simulink model "accelerationTestUnit"  (R2015b)
settings: Solver=FixedStepAuto  StartTime=0.0  StopTime=inf  RelTol=1e-3
undefined symbols (not defined in the file): DiscIntNeverNeededParam
libraries: frdmtfcshieldlib x2, freescalecupcompanionlib x1, simulink_extras x1
settings Model: SimulationMode=external  ExtModeTrigDuration=125  ExtModeArchiveMode=auto  ExtModeArchiveFileName=data-measures  ExtModeArchiveDirName=C:\Users\ap6515\Desktop\Group Project  ExtModeAddSuffixToVar=on  ExtModeWriteAllDataToWs=on  Creator=DM1515  LastModifiedBy=ap6515
settings OptimizationCC: OptimizeModelRefInitCode=on  LifeSpan=1  MaxStackSize=64
settings HardwareCC: ProdBitPerPointer=32  ProdLargestAtomicInteger=Long  ProdLargestAtomicFloat=Double  ProdWordSize=32  ProdHWDeviceType=ARM Compatible->ARM Cortex
settings RTWCC: SystemTargetFile=ert.tlc  TemplateMakefile=ert_default_tmf  Description=Embedded Coder  Toolchain=GNU Tools for ARM Embedded Processors
settings CodeAppCC: IgnoreCustomStorageClasses=off

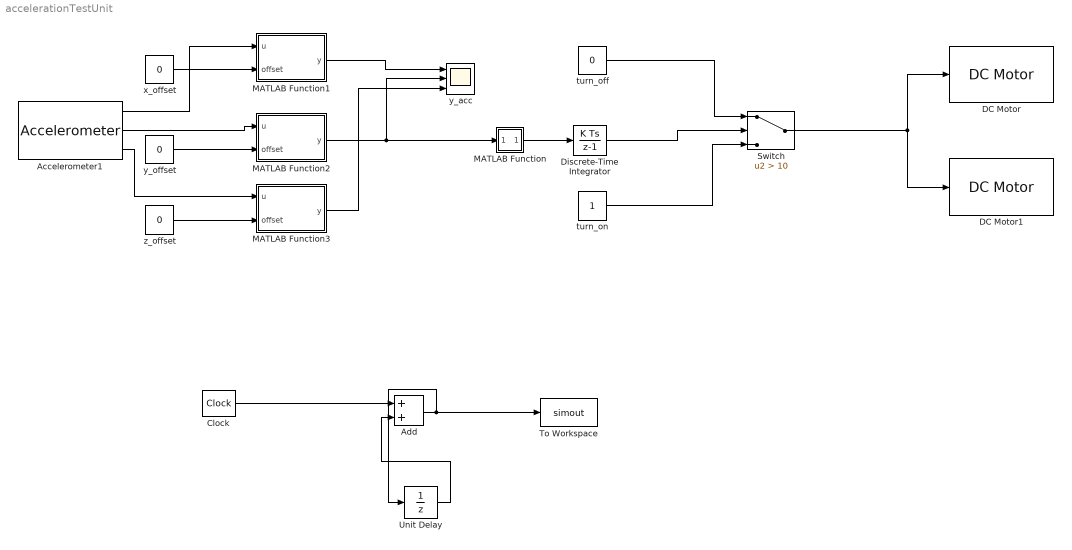
== system accelerationTestUnit ==
  Accelerometer1 : freescalecupcompanionlib/Accelerometer  SampleTime=-1
  Add : Sum
  Clock : simulink_extras/Flip Flops/Clock  period=2
  DC Motor : frdmtfcshieldlib/DC Motor  WhichMotor=A
  DC Motor1 : frdmtfcshieldlib/DC Motor  WhichMotor=B
  Discrete-Time Integrator : DiscreteIntegrator  InitialConditionSetting=State (most efficient)  SampleTime=-1  ICPrevOutput=DiscIntNeverNeededParam  ICPrevScaledInput=DiscIntNeverNeededParam
  MATLAB Function : MATLAB Function  TreatAsAtomicUnit=on
  MATLAB Function1 : MATLAB Function  TreatAsAtomicUnit=on
  MATLAB Function2 : MATLAB Function  TreatAsAtomicUnit=on
  MATLAB Function3 : MATLAB Function  TreatAsAtomicUnit=on
  Switch : Switch  Criteria=u2 > Threshold  Threshold=10
  To Workspace : ToWorkspace  VariableName=simout  SaveFormat=Structure With Time  SampleTime=-1
  Unit Delay : UnitDelay  SampleTime=-1
  turn_off : Constant  Value=0  SampleTime=-1
  turn_on : Constant  SampleTime=-1
  x_offset : Constant  Value=0  SampleTime=-1
  y_acc : Scope  NumInputPorts=3
  y_offset : Constant  Value=0  SampleTime=-1
  z_offset : Constant  Value=0  SampleTime=-1
  wires:
  Switch/1 -> DC Motor/1, DC Motor1/1
  turn_off/1 -> Switch/1
  turn_on/1 -> Switch/3
  Discrete-Time Integrator/1 -> Switch/2
  MATLAB Function/1(y) -> Discrete-Time Integrator/1
  Accelerometer1/1 -> MATLAB Function1/1(u)
  Accelerometer1/2 -> MATLAB Function2/1(u)
  MATLAB Function2/1(y) -> y_acc/2, MATLAB Function/1(u)
  x_offset/1 -> MATLAB Function1/2(offset)
  Accelerometer1/3 -> MATLAB Function3/1(u)
  y_offset/1 -> MATLAB Function2/2(offset)
  z_offset/1 -> MATLAB Function3/2(offset)
  Clock/1 -> Add/1
  Unit Delay/1 -> Add/2
  Add/1 -> To Workspace/1, Unit Delay/1
  MATLAB Function1/1(y) -> y_acc/1
  MATLAB Function3/1(y) -> y_acc/3

== matlab function accelerationTestUnit/MATLAB Function1 ==
  data: u input; y output; offset input
function y = fcn(u, offset)
%#codegen

y = u - offset;

== matlab function accelerationTestUnit/MATLAB Function ==
  data: u input; y output
function y = fcn(u)
%#codegen

y = u*9.81;

== matlab function accelerationTestUnit/MATLAB Function2 ==
  data: u input; y output; offset input
function y = fcn(u, offset)
%#codegen

y = u - offset;

== matlab function accelerationTestUnit/MATLAB Function3 ==
  data: u input; y output; offset input
function y = fcn(u, offset)
%#codegen

y = u - offset;
